simulink model "swim_12B_with_contracts_PP"  (R2019b)
settings: Solver=FixedStepDiscrete  StartTime=0.0  StopTime=10.0  FixedStep=0.200000  RelTol=1e-3  EnableMultiTasking=on
model workspace (MAT data in the model file):
  ContractValidatorBlocksMap = containers.Map
  ContractValidatorBlocksMap.serialization.keys = {'swim_12B_with_contracts/swim_12B_SWIMSpec/validator'}
  ContractValidatorBlocksMap.serialization.values{1}.block = 'swim_12B_with_contracts/swim_12B_SWIMSpec/validator'
  ContractValidatorBlocksMap.serialization.values{1}.assumePorts = 1
  ContractValidatorBlocksMap.serialization.values{1}.guaranteePorts = 3
  ContractValidatorBlocksMap.serialization.values{1}.modeBlocksPorts = 0
  ContractValidatorBlocksMap.serialization.values{1}.portHandles.Inport = [713.000976562 714.000976562 715.000976562 716.000976562]
  ContractValidatorBlocksMap.serialization.values{1}.portHandles.Outport = 717.000976562
  ContractValidatorBlocksMap.serialization.values{1}.portHandles.Enable = []
  ContractValidatorBlocksMap.serialization.values{1}.portHandles.Trigger = []
  ContractValidatorBlocksMap.serialization.values{1}.portHandles.State = []
  ContractValidatorBlocksMap.serialization.values{1}.portHandles.LConn = []
  ContractValidatorBlocksMap.serialization.values{1}.portHandles.RConn = []
  ContractValidatorBlocksMap.serialization.values{1}.portHandles.Ifaction = []
  ContractValidatorBlocksMap.serialization.values{1}.portHandles.Reset = []
  ContractValidatorBlocksMap.serialization.values{1}.portConnectivity(1).Type = '1'
  ContractValidatorBlocksMap.serialization.values{1}.portConnectivity(1).Position = [1210 730]
  ContractValidatorBlocksMap.serialization.values{1}.portConnectivity(1).SrcBlock = 336.034667969
  ContractValidatorBlocksMap.serialization.values{1}.portConnectivity(1).SrcPort = 0
  ContractValidatorBlocksMap.serialization.values{1}.portConnectivity(1).DstBlock = []
  ContractValidatorBlocksMap.serialization.values{1}.portConnectivity(1).DstPort = []
  ContractValidatorBlocksMap.serialization.values{1}.portConnectivity(2).Type = '2'
  ContractValidatorBlocksMap.serialization.values{1}.portConnectivity(2).Position = [1210 775]
  ContractValidatorBlocksMap.serialization.values{1}.portConnectivity(2).SrcBlock = 340.034667969
  ContractValidatorBlocksMap.serialization.values{1}.portConnectivity(2).SrcPort = 0
  ContractValidatorBlocksMap.serialization.values{1}.portConnectivity(2).DstBlock = []
  ContractValidatorBlocksMap.serialization.values{1}.portConnectivity(2).DstPort = []
  ContractValidatorBlocksMap.serialization.values{1}.portConnectivity(3).Type = '3'
  ContractValidatorBlocksMap.serialization.values{1}.portConnectivity(3).Position = [1210 820]
  ContractValidatorBlocksMap.serialization.values{1}.portConnectivity(3).SrcBlock = 344.034667969
  ContractValidatorBlocksMap.serialization.values{1}.portConnectivity(3).SrcPort = 0
  ContractValidatorBlocksMap.serialization.values{1}.portConnectivity(3).DstBlock = []
  ContractValidatorBlocksMap.serialization.values{1}.portConnectivity(3).DstPort = []
  ContractValidatorBlocksMap.serialization.values{1}.portConnectivity(4).Type = '4'
  ContractValidatorBlocksMap.serialization.values{1}.portConnectivity(4).Position = [1210 865]
  ContractValidatorBlocksMap.serialization.values{1}.portConnectivity(4).SrcBlock = 348.034667969
  ContractValidatorBlocksMap.serialization.values{1}.portConnectivity(4).SrcPort = 0
  ContractValidatorBlocksMap.serialization.values{1}.portConnectivity(4).DstBlock = []
  ContractValidatorBlocksMap.serialization.values{1}.portConnectivity(4).DstPort = []
  ContractValidatorBlocksMap.serialization.values{1}.portConnectivity(5).Type = '1'
  ContractValidatorBlocksMap.serialization.values{1}.portConnectivity(5).Position = [1250 800]
  ContractValidatorBlocksMap.serialization.values{1}.portConnectivity(5).SrcBlock = []
  ContractValidatorBlocksMap.serialization.values{1}.portConnectivity(5).SrcPort = []
  ContractValidatorBlocksMap.serialization.values{1}.portConnectivity(5).DstBlock = 379.034667969
  ContractValidatorBlocksMap.serialization.values{1}.portConnectivity(5).DstPort = 0
  ContractValidatorBlocksMap.serialization.uniformity = 0
  ContractValidatorBlocksMap.serialization.keyType = 'char'
  ContractValidatorBlocksMap.serialization.valueType = 'any'
  already_pp = 1
  compositionalMap.analysisNames = {'swim_12B_with_contracts_PP/swim_airspeed'}
  compositionalMap.compositionalOptions = {{''}}
  compositionalMap.selectedOptions = 1
  maskControlsMap = containers.Map
  maskControlsMap.serialization.keys = {'swim_12B_with_contracts_PP/swim_12B_SWIMSpec/SWIM_minus_002'}
  maskControlsMap.serialization.values = {{'Display_counter_example_as_signals', 'Display_counter_example_as_tables', 'Display_counter_example_as_HTML_tables', 'Generate_an_outer_model_for_the_counter_example', 'Generate_an_inner_model_for_the_counter_example'}}
  maskControlsMap.serialization.uniformity = 0
  maskControlsMap.serialization.keyType = 'char'
  maskControlsMap.serialization.valueType = 'any'
  nodeNameToBlockNameMap = containers.Map
  nodeNameToBlockNameMap.serialization.keys{1} = 'A_1'
  nodeNameToBlockNameMap.serialization.keys{2} = 'A_equal__equal__gt_B_1'
  nodeNameToBlockNameMap.serialization.keys{3} = 'AircraftWeight_lbs_1'
  nodeNameToBlockNameMap.serialization.keys{4} = 'AirspeedMonitoring_1'
  nodeNameToBlockNameMap.serialization.keys{5} = 'AirspeedMonitoring_435_035'
  nodeNameToBlockNameMap.serialization.keys{6} = 'B_1'
  nodeNameToBlockNameMap.serialization.keys{7} = 'CalculateminimumimpactpressureforAGCASoperationtobesuspendedandsenttostandby_1'
  nodeNameToBlockNameMap.serialization.keys{8} = 'CalculateminimumimpactpressureforAGCASoperationtobesuspendedandsenttostandby_495_035'
  nodeNameToBlockNameMap.serialization.keys{9} = 'CalculateminimumimpactpressureforwarningtopilotthatAGCASoperationisdegraded_1'
  nodeNameToBlockNameMap.serialization.keys{10} = 'CalculateminimumimpactpressureforwarningtopilotthatAGCASoperationisdegraded_503_035'
  nodeNameToBlockNameMap.serialization.keys{11} = 'CalculatetheminimumcalibratedairspeedbasedonCatSwitch_1'
  nodeNameToBlockNameMap.serialization.keys{12} = 'CalculatetheminimumcalibratedairspeedbasedonCatSwitch_519_002'
  nodeNameToBlockNameMap.serialization.keys{13} = 'Constant1_1'
  nodeNameToBlockNameMap.serialization.keys{14} = 'Constant2_1'
  nodeNameToBlockNameMap.serialization.keys{15} = 'Constant3_1'
  nodeNameToBlockNameMap.serialization.keys{16} = 'Constant4_1'
  nodeNameToBlockNameMap.serialization.keys{17} = 'Constant_1'
  nodeNameToBlockNameMap.serialization.keys{18} = 'E_AI_IMPACT_PRESSURE_1'
  nodeNameToBlockNameMap.serialization.keys{19} = 'Gain1_1'
  nodeNameToBlockNameMap.serialization.keys{20} = 'Gain_1'
  nodeNameToBlockNameMap.serialization.keys{21} = 'Gettheaircraftweight_1'
  nodeNameToBlockNameMap.serialization.keys{22} = 'Gettheaircraftweight_566_001'
  nodeNameToBlockNameMap.serialization.keys{23} = 'If1_1'
  nodeNameToBlockNameMap.serialization.keys{24} = 'If1_2'
  nodeNameToBlockNameMap.serialization.keys{25} = 'IfActionSubsystem1_1'
  nodeNameToBlockNameMap.serialization.keys{26} = 'IfActionSubsystem1_447_035'
  nodeNameToBlockNameMap.serialization.keys{27} = 'IfActionSubsystem1_537_018'
  nodeNameToBlockNameMap.serialization.keys{28} = 'IfActionSubsystem1_592_001'
  nodeNameToBlockNameMap.serialization.keys{29} = 'IfActionSubsystem1_608_001'
  nodeNameToBlockNameMap.serialization.keys{30} = 'IfActionSubsystem2_1'
  nodeNameToBlockNameMap.serialization.keys{31} = 'IfActionSubsystem2_452_035'
  nodeNameToBlockNameMap.serialization.keys{32} = 'IfActionSubsystem3_1'
  nodeNameToBlockNameMap.serialization.keys{33} = 'IfActionSubsystem3_457_035'
  nodeNameToBlockNameMap.serialization.keys{34} = 'IfActionSubsystem_1'
  nodeNameToBlockNameMap.serialization.keys{35} = 'IfActionSubsystem_442_035'
  nodeNameToBlockNameMap.serialization.keys{36} = 'IfActionSubsystem_524_002'
  nodeNameToBlockNameMap.serialization.keys{37} = 'IfActionSubsystem_582_001'
  nodeNameToBlockNameMap.serialization.keys{38} = 'IfActionSubsystem_587_001'
  nodeNameToBlockNameMap.serialization.keys{39} = 'If_1'
  nodeNameToBlockNameMap.serialization.keys{40} = 'If_2'
  nodeNameToBlockNameMap.serialization.keys{41} = 'In1_1'
  nodeNameToBlockNameMap.serialization.keys{42} = 'IssueWarning_1'
  nodeNameToBlockNameMap.serialization.keys{43} = 'IssueWarning_570_001'
  nodeNameToBlockNameMap.serialization.keys{44} = 'LogicalOperator1_1'
  nodeNameToBlockNameMap.serialization.keys{45} = 'LogicalOperator2_1'
  nodeNameToBlockNameMap.serialization.keys{46} = 'LogicalOperator_1'
  nodeNameToBlockNameMap.serialization.keys{47} = 'Logical_newline_Operator1_1'
  nodeNameToBlockNameMap.serialization.keys{48} = 'Logical_newline_Operator_1'
  nodeNameToBlockNameMap.serialization.keys{49} = 'Merge1_1'
  nodeNameToBlockNameMap.serialization.keys{50} = 'Merge_1'
  nodeNameToBlockNameMap.serialization.keys{51} = 'Out1_1'
  nodeNameToBlockNameMap.serialization.keys{52} = 'RelationalOperator1_1'
  nodeNameToBlockNameMap.serialization.keys{53} = 'RelationalOperator2_1'
  nodeNameToBlockNameMap.serialization.keys{54} = 'RelationalOperator3_1'
  nodeNameToBlockNameMap.serialization.keys{55} = 'RelationalOperator4_1'
  nodeNameToBlockNameMap.serialization.keys{56} = 'RelationalOperator_1'
  nodeNameToBlockNameMap.serialization.keys{57} = 'SWIMSpec_CalAirspeedMin_1'
  nodeNameToBlockNameMap.serialization.keys{58} = 'SWIMSpec_lowSpeedWarningAllowed_1'
  nodeNameToBlockNameMap.serialization.keys{59} = 'SWIMSpec_storeCat_1'
  nodeNameToBlockNameMap.serialization.keys{60} = 'SWIMSpec_swimGet_agcasLowSpeedWarn_1'
  nodeNameToBlockNameMap.serialization.keys{61} = 'SWIMSpec_vehAirPress_1'
  nodeNameToBlockNameMap.serialization.keys{62} = 'SWIMSpec_warningTrigForMinPress_1'
  nodeNameToBlockNameMap.serialization.keys{63} = 'SWIMSpec_weight_1'
  nodeNameToBlockNameMap.serialization.keys{64} = 'SWIM_ASWarningAllowed_1'
  nodeNameToBlockNameMap.serialization.keys{65} = 'SWIM_AirspeedWarningAllowed_1'
  nodeNameToBlockNameMap.serialization.keys{66} = 'SWIM_CalAirspeedmin_kts_1'
  nodeNameToBlockNameMap.serialization.keys{67} = 'SWIM_Qcmin_lbspft2_1'
  nodeNameToBlockNameMap.serialization.keys{68} = 'SWIM_SelfAgcasLowSpeedWarn_1'
  nodeNameToBlockNameMap.serialization.keys{69} = 'SWIM_minus_001A_1'
  nodeNameToBlockNameMap.serialization.keys{70} = 'SWIM_minus_001A_340_035'
  nodeNameToBlockNameMap.serialization.keys{71} = 'SWIM_minus_001B_1'
  nodeNameToBlockNameMap.serialization.keys{72} = 'SWIM_minus_001B_344_035'
  nodeNameToBlockNameMap.serialization.keys{73} = 'SWIM_minus_002_1'
  nodeNameToBlockNameMap.serialization.keys{74} = 'SWIM_minus_002_348_035'
  nodeNameToBlockNameMap.serialization.keys{75} = 'S_ImpactPressure_lbspft2_1'
  nodeNameToBlockNameMap.serialization.keys{76} = 'Sqrt_1'
  nodeNameToBlockNameMap.serialization.keys{77} = 'Sum1_1'
  nodeNameToBlockNameMap.serialization.keys{78} = 'Sum_1'
  nodeNameToBlockNameMap.serialization.keys{79} = 'UnitDelay_1'
  nodeNameToBlockNameMap.serialization.keys{80} = 'assume_1'
  nodeNameToBlockNameMap.serialization.keys{81} = 'assume_336_035'
  nodeNameToBlockNameMap.serialization.keys{82} = 'cvGet_V_AgcasLowSpeedWarn_1'
  nodeNameToBlockNameMap.serialization.keys{83} = 'diGet_S_CatSwitchPosition_1'
  nodeNameToBlockNameMap.serialization.keys{84} = 'diGet_S_LandingGearAltFlap_1'
  nodeNameToBlockNameMap.serialization.keys{85} = 'guarantee_1'
  nodeNameToBlockNameMap.serialization.keys{86} = 'lowSpeedWarningTrue_operator_1'
  nodeNameToBlockNameMap.serialization.keys{87} = 'muxGet_T_Mux_AircraftGrossWeight_lbs_1'
  nodeNameToBlockNameMap.serialization.keys{88} = 'muxGet_T_Mux_AirspeedMonitorEnable_1'
  nodeNameToBlockNameMap.serialization.keys{89} = 'o_SWIM_CalAirspeedmin_kts_1'
  nodeNameToBlockNameMap.serialization.keys{90} = 'o_SWIM_QcMinDisable_lbspft2_1'
  nodeNameToBlockNameMap.serialization.keys{91} = 'o_SWIM_Qcmin_lbspft2_1'
  nodeNameToBlockNameMap.serialization.keys{92} = 'olcGet_AgcasInterlocks_1'
  nodeNameToBlockNameMap.serialization.keys{93} = 'spec122_operator_1'
  nodeNameToBlockNameMap.serialization.keys{94} = 'spec122_rhs_2_1'
  nodeNameToBlockNameMap.serialization.keys{95} = 'spec139_operator_1'
  nodeNameToBlockNameMap.serialization.keys{96} = 'spec139_operator_355_035'
  nodeNameToBlockNameMap.serialization.keys{97} = 'spec156_operator_1'
  nodeNameToBlockNameMap.serialization.keys{98} = 'spec156_operator_356_035'
  nodeNameToBlockNameMap.serialization.keys{99} = 'spec170_operator_1'
  nodeNameToBlockNameMap.serialization.keys{100} = 'spec170_operator_357_035'
  nodeNameToBlockNameMap.serialization.keys{101} = 'sqrtOfWeight_sqrt_call_1'
  nodeNameToBlockNameMap.serialization.keys{102} = 'swimGet_AgcasLowSpeedWarn_1'
  nodeNameToBlockNameMap.serialization.keys{103} = 'swimGet_QcMinDisable_lbspft2_1'
  nodeNameToBlockNameMap.serialization.keys{104} = 'swim_12B_SWIMSpec_328_035'
  nodeNameToBlockNameMap.serialization.keys{105} = 'swim_12B_with_contracts_PP'
  nodeNameToBlockNameMap.serialization.keys{106} = 'swim_airspeed_1'
  nodeNameToBlockNameMap.serialization.keys{107} = 'swim_airspeed_2'
  nodeNameToBlockNameMap.serialization.keys{108} = 'swim_airspeed_3'
  nodeNameToBlockNameMap.serialization.keys{109} = 'swim_airspeed_4'
  nodeNameToBlockNameMap.serialization.keys{110} = 'swim_airspeed_427_035'
  nodeNameToBlockNameMap.serialization.keys{111} = 'swim_airspeed_5'
  nodeNameToBlockNameMap.serialization.keys{112} = 'valid_1'
  nodeNameToBlockNameMap.serialization.keys{113} = 'xxSWIMSpec_10_operator_1'
  nodeNameToBlockNameMap.serialization.keys{114} = 'xxSWIMSpec_11_operator_1'
  nodeNameToBlockNameMap.serialization.keys{115} = 'xxSWIMSpec_12_rhs_1'
  nodeNameToBlockNameMap.serialization.keys{116} = 'xxSWIMSpec_13_rhs_1'
  nodeNameToBlockNameMap.serialization.keys{117} = 'xxSWIMSpec_14_rhs_1'
  nodeNameToBlockNameMap.serialization.keys{118} = 'xxSWIMSpec_1_operator_1'
  nodeNameToBlockNameMap.serialization.keys{119} = 'xxSWIMSpec_2_operator_1'
  nodeNameToBlockNameMap.serialization.keys{120} = 'xxSWIMSpec_2_rhs_2_1'
  nodeNameToBlockNameMap.serialization.keys{121} = 'xxSWIMSpec_3_operator_1'
  nodeNameToBlockNameMap.serialization.keys{122} = 'xxSWIMSpec_4_operator_1'
  nodeNameToBlockNameMap.serialization.keys{123} = 'xxSWIMSpec_4_rhs_1_1'
  nodeNameToBlockNameMap.serialization.keys{124} = 'xxSWIMSpec_5_operator_1'
  nodeNameToBlockNameMap.serialization.keys{125} = 'xxSWIMSpec_5_rhs_2_1'
  nodeNameToBlockNameMap.serialization.keys{126} = 'xxSWIMSpec_6_operator_1'
  nodeNameToBlockNameMap.serialization.keys{127} = 'xxSWIMSpec_7_operator_1'
  nodeNameToBlockNameMap.serialization.keys{128} = 'xxSWIMSpec_8_operator_1'
  nodeNameToBlockNameMap.serialization.keys{129} = 'xxSWIMSpec_8_rhs_1_1'
  nodeNameToBlockNameMap.serialization.keys{130} = 'xxSWIMSpec_9_operator_1'
  nodeNameToBlockNameMap.serialization.keys{131} = 'xxSWIMSpec_9_rhs_2_1'
  nodeNameToBlockNameMap.serialization.values{1} = 'swim_12B_with_contracts_PP/swim_12B_SWIMSpec/spec170_operator/A'
  nodeNameToBlockNameMap.serialization.values{2} = 'swim_12B_with_contracts_PP/swim_12B_SWIMSpec/spec170_operator/A_equal__equal__gt_B'
  nodeNameToBlockNameMap.serialization.values{3} = 'swim_12B_with_contracts_PP/swim_airspeed/Gettheaircraftweight/AircraftWeight_lbs'
  nodeNameToBlockNameMap.serialization.values{4} = 'swim_12B_with_contracts_PP/swim_airspeed/AirspeedMonitoring'
  nodeNameToBlockNameMap.serialization.values{5} = 'swim_12B_with_contracts_PP/swim_airspeed/AirspeedMonitoring'
  nodeNameToBlockNameMap.serialization.values{6} = 'swim_12B_with_contracts_PP/swim_12B_SWIMSpec/spec170_operator/B'
  nodeNameToBlockNameMap.serialization.values{7} = 'swim_12B_with_contracts_PP/swim_airspeed/CalculateminimumimpactpressureforAGCASoperationtobesuspendedandsenttostandby'
  nodeNameToBlockNameMap.serialization.values{8} = 'swim_12B_with_contracts_PP/swim_airspeed/CalculateminimumimpactpressureforAGCASoperationtobesuspendedandsenttostandby'
  nodeNameToBlockNameMap.serialization.values{9} = 'swim_12B_with_contracts_PP/swim_airspeed/CalculateminimumimpactpressureforwarningtopilotthatAGCASoperationisdegraded'
  nodeNameToBlockNameMap.serialization.values{10} = 'swim_12B_with_contracts_PP/swim_airspeed/CalculateminimumimpactpressureforwarningtopilotthatAGCASoperationisdegraded'
  nodeNameToBlockNameMap.serialization.values{11} = 'swim_12B_with_contracts_PP/swim_airspeed/CalculatetheminimumcalibratedairspeedbasedonCatSwitch'
  nodeNameToBlockNameMap.serialization.values{12} = 'swim_12B_with_contracts_PP/swim_airspeed/CalculatetheminimumcalibratedairspeedbasedonCatSwitch'
  nodeNameToBlockNameMap.serialization.values{13} = 'swim_12B_with_contracts_PP/swim_airspeed/IssueWarning/Constant1'
  nodeNameToBlockNameMap.serialization.values{14} = 'swim_12B_with_contracts_PP/swim_airspeed/IssueWarning/Constant2'
  nodeNameToBlockNameMap.serialization.values{15} = 'swim_12B_with_contracts_PP/swim_airspeed/IssueWarning/Constant3'
  nodeNameToBlockNameMap.serialization.values{16} = 'swim_12B_with_contracts_PP/swim_airspeed/IssueWarning/Constant4'
  nodeNameToBlockNameMap.serialization.values{17} = 'swim_12B_with_contracts_PP/swim_airspeed/IssueWarning/IfActionSubsystem/IfActionSubsystem1/Constant'
  nodeNameToBlockNameMap.serialization.values{18} = 'swim_12B_with_contracts_PP/E_AI_IMPACT_PRESSURE'
  nodeNameToBlockNameMap.serialization.values{19} = 'swim_12B_with_contracts_PP/swim_airspeed/CalculateminimumimpactpressureforwarningtopilotthatAGCASoperationisdegraded/Gain1'
  nodeNameToBlockNameMap.serialization.values{20} = 'swim_12B_with_contracts_PP/swim_airspeed/CalculatetheminimumcalibratedairspeedbasedonCatSwitch/IfActionSubsystem1/Gain'
  nodeNameToBlockNameMap.serialization.values{21} = 'swim_12B_with_contracts_PP/swim_airspeed/Gettheaircraftweight'
  nodeNameToBlockNameMap.serialization.values{22} = 'swim_12B_with_contracts_PP/swim_airspeed/Gettheaircraftweight'
  nodeNameToBlockNameMap.serialization.values{23} = 'swim_12B_with_contracts_PP/swim_airspeed/AirspeedMonitoring/If1'
  nodeNameToBlockNameMap.serialization.values{24} = 'swim_12B_with_contracts_PP/swim_airspeed/AirspeedMonitoring/If1'
  nodeNameToBlockNameMap.serialization.values{25} = 'swim_12B_with_contracts_PP/swim_airspeed/IssueWarning/IfActionSubsystem1'
  nodeNameToBlockNameMap.serialization.values{26} = 'swim_12B_with_contracts_PP/swim_airspeed/AirspeedMonitoring/IfActionSubsystem1'
  nodeNameToBlockNameMap.serialization.values{27} = 'swim_12B_with_contracts_PP/swim_airspeed/CalculatetheminimumcalibratedairspeedbasedonCatSwitch/IfActionSubsystem1'
  nodeNameToBlockNameMap.serialization.values{28} = 'swim_12B_with_contracts_PP/swim_airspeed/IssueWarning/IfActionSubsystem/IfActionSubsystem1'
  nodeNameToBlockNameMap.serialization.values{29} = 'swim_12B_with_contracts_PP/swim_airspeed/IssueWarning/IfActionSubsystem1'
  nodeNameToBlockNameMap.serialization.values{30} = 'swim_12B_with_contracts_PP/swim_airspeed/AirspeedMonitoring/IfActionSubsystem2'
  nodeNameToBlockNameMap.serialization.values{31} = 'swim_12B_with_contracts_PP/swim_airspeed/AirspeedMonitoring/IfActionSubsystem2'
  nodeNameToBlockNameMap.serialization.values{32} = 'swim_12B_with_contracts_PP/swim_airspeed/AirspeedMonitoring/IfActionSubsystem3'
  nodeNameToBlockNameMap.serialization.values{33} = 'swim_12B_with_contracts_PP/swim_airspeed/AirspeedMonitoring/IfActionSubsystem3'
  nodeNameToBlockNameMap.serialization.values{34} = 'swim_12B_with_contracts_PP/swim_airspeed/IssueWarning/IfActionSubsystem'
  nodeNameToBlockNameMap.serialization.values{35} = 'swim_12B_with_contracts_PP/swim_airspeed/AirspeedMonitoring/IfActionSubsystem'
  nodeNameToBlockNameMap.serialization.values{36} = 'swim_12B_with_contracts_PP/swim_airspeed/CalculatetheminimumcalibratedairspeedbasedonCatSwitch/IfActionSubsystem'
  nodeNameToBlockNameMap.serialization.values{37} = 'swim_12B_with_contracts_PP/swim_airspeed/IssueWarning/IfActionSubsystem'
  nodeNameToBlockNameMap.serialization.values{38} = 'swim_12B_with_contracts_PP/swim_airspeed/IssueWarning/IfActionSubsystem/IfActionSubsystem'
  nodeNameToBlockNameMap.serialization.values{39} = 'swim_12B_with_contracts_PP/swim_airspeed/IssueWarning/If'
  nodeNameToBlockNameMap.serialization.values{40} = 'swim_12B_with_contracts_PP/swim_airspeed/IssueWarning/If'
  nodeNameToBlockNameMap.serialization.values{41} = 'swim_12B_with_contracts_PP/swim_airspeed/IssueWarning/IfActionSubsystem1/In1'
  nodeNameToBlockNameMap.serialization.values{42} = 'swim_12B_with_contracts_PP/swim_airspeed/IssueWarning'
  nodeNameToBlockNameMap.serialization.values{43} = 'swim_12B_with_contracts_PP/swim_airspeed/IssueWarning'
  nodeNameToBlockNameMap.serialization.values{44} = 'swim_12B_with_contracts_PP/swim_airspeed/IssueWarning/LogicalOperator1'
  nodeNameToBlockNameMap.serialization.values{45} = 'swim_12B_with_contracts_PP/swim_airspeed/IssueWarning/LogicalOperator2'
  nodeNameToBlockNameMap.serialization.values{46} = 'swim_12B_with_contracts_PP/swim_airspeed/AirspeedMonitoring/LogicalOperator'
  nodeNameToBlockNameMap.serialization.values{47} = 'swim_12B_with_contracts_PP/swim_12B_SWIMSpec/spec170_operator/Logical_newline_Operator1'
  nodeNameToBlockNameMap.serialization.values{48} = 'swim_12B_with_contracts_PP/swim_12B_SWIMSpec/spec170_operator/Logical_newline_Operator'
  nodeNameToBlockNameMap.serialization.values{49} = 'swim_12B_with_contracts_PP/swim_airspeed/AirspeedMonitoring/Merge1'
  nodeNameToBlockNameMap.serialization.values{50} = 'swim_12B_with_contracts_PP/swim_airspeed/IssueWarning/Merge'
  nodeNameToBlockNameMap.serialization.values{51} = 'swim_12B_with_contracts_PP/swim_airspeed/IssueWarning/IfActionSubsystem1/Out1'
  nodeNameToBlockNameMap.serialization.values{52} = 'swim_12B_with_contracts_PP/swim_airspeed/IssueWarning/RelationalOperator1'
  nodeNameToBlockNameMap.serialization.values{53} = 'swim_12B_with_contracts_PP/swim_airspeed/IssueWarning/RelationalOperator2'
  nodeNameToBlockNameMap.serialization.values{54} = 'swim_12B_with_contracts_PP/swim_airspeed/IssueWarning/RelationalOperator3'
  nodeNameToBlockNameMap.serialization.values{55} = 'swim_12B_with_contracts_PP/swim_airspeed/IssueWarning/RelationalOperator4'
  nodeNameToBlockNameMap.serialization.values{56} = 'swim_12B_with_contracts_PP/swim_airspeed/IssueWarning/IfActionSubsystem/RelationalOperator'
  nodeNameToBlockNameMap.serialization.values{57} = 'swim_12B_with_contracts_PP/swim_12B_SWIMSpec/SWIMSpec_CalAirspeedMin'
  nodeNameToBlockNameMap.serialization.values{58} = 'swim_12B_with_contracts_PP/swim_12B_SWIMSpec/SWIMSpec_lowSpeedWarningAllowed'
  nodeNameToBlockNameMap.serialization.values{59} = 'swim_12B_with_contracts_PP/swim_12B_SWIMSpec/SWIMSpec_storeCat'
  nodeNameToBlockNameMap.serialization.values{60} = 'swim_12B_with_contracts_PP/swim_12B_SWIMSpec/SWIMSpec_swimGet_agcasLowSpeedWarn'
  nodeNameToBlockNameMap.serialization.values{61} = 'swim_12B_with_contracts_PP/swim_12B_SWIMSpec/SWIMSpec_vehAirPress'
  nodeNameToBlockNameMap.serialization.values{62} = 'swim_12B_with_contracts_PP/swim_12B_SWIMSpec/SWIMSpec_warningTrigForMinPress'
  nodeNameToBlockNameMap.serialization.values{63} = 'swim_12B_with_contracts_PP/swim_12B_SWIMSpec/SWIMSpec_weight'
  nodeNameToBlockNameMap.serialization.values{64} = 'swim_12B_with_contracts_PP/SWIM_ASWarningAllowed'
  nodeNameToBlockNameMap.serialization.values{65} = 'swim_12B_with_contracts_PP/swim_airspeed/IssueWarning/SWIM_AirspeedWarningAllowed'
  nodeNameToBlockNameMap.serialization.values{66} = 'swim_12B_with_contracts_PP/SWIM_CalAirspeedmin_kts'
  nodeNameToBlockNameMap.serialization.values{67} = 'swim_12B_with_contracts_PP/SWIM_Qcmin_lbspft2'
  nodeNameToBlockNameMap.serialization.values{68} = 'swim_12B_with_contracts_PP/swim_airspeed/IssueWarning/SWIM_SelfAgcasLowSpeedWarn'
  nodeNameToBlockNameMap.serialization.values{69} = 'swim_12B_with_contracts_PP/swim_12B_SWIMSpec/SWIM_minus_001A'
  nodeNameToBlockNameMap.serialization.values{70} = 'swim_12B_with_contracts_PP/swim_12B_SWIMSpec/SWIM_minus_001A'
  nodeNameToBlockNameMap.serialization.values{71} = 'swim_12B_with_contracts_PP/swim_12B_SWIMSpec/SWIM_minus_001B'
  nodeNameToBlockNameMap.serialization.values{72} = 'swim_12B_with_contracts_PP/swim_12B_SWIMSpec/SWIM_minus_001B'
  nodeNameToBlockNameMap.serialization.values{73} = 'swim_12B_with_contracts_PP/swim_12B_SWIMSpec/SWIM_minus_002'
  nodeNameToBlockNameMap.serialization.values{74} = 'swim_12B_with_contracts_PP/swim_12B_SWIMSpec/SWIM_minus_002'
  nodeNameToBlockNameMap.serialization.values{75} = 'swim_12B_with_contracts_PP/swim_airspeed/IssueWarning/S_ImpactPressure_lbspft2'
  nodeNameToBlockNameMap.serialization.values{76} = 'swim_12B_with_contracts_PP/swim_airspeed/CalculatetheminimumcalibratedairspeedbasedonCatSwitch/IfActionSubsystem1/Sqrt'
  nodeNameToBlockNameMap.serialization.values{77} = 'swim_12B_with_contracts_PP/swim_airspeed/CalculateminimumimpactpressureforwarningtopilotthatAGCASoperationisdegraded/Sum1'
  nodeNameToBlockNameMap.serialization.values{78} = 'swim_12B_with_contracts_PP/swim_airspeed/CalculatetheminimumcalibratedairspeedbasedonCatSwitch/IfActionSubsystem1/Sum'
  nodeNameToBlockNameMap.serialization.values{79} = 'swim_12B_with_contracts_PP/swim_airspeed/IssueWarning/UnitDelay'
  nodeNameToBlockNameMap.serialization.values{80} = 'swim_12B_with_contracts_PP/swim_12B_SWIMSpec/assume'
  nodeNameToBlockNameMap.serialization.values{81} = 'swim_12B_with_contracts_PP/swim_12B_SWIMSpec/assume'
  nodeNameToBlockNameMap.serialization.values{82} = 'swim_12B_with_contracts_PP/cvGet_V_AgcasLowSpeedWarn'
  nodeNameToBlockNameMap.serialization.values{83} = 'swim_12B_with_contracts_PP/diGet_S_CatSwitchPosition'
  nodeNameToBlockNameMap.serialization.values{84} = 'swim_12B_with_contracts_PP/diGet_S_LandingGearAltFlap'
  nodeNameToBlockNameMap.serialization.values{85} = 'swim_12B_with_contracts_PP/swim_12B_SWIMSpec/SWIM_minus_002/guarantee'
  nodeNameToBlockNameMap.serialization.values{86} = 'swim_12B_with_contracts_PP/swim_12B_SWIMSpec/lowSpeedWarningTrue_operator'
  nodeNameToBlockNameMap.serialization.values{87} = 'swim_12B_with_contracts_PP/muxGet_T_Mux_AircraftGrossWeight_lbs'
  nodeNameToBlockNameMap.serialization.values{88} = 'swim_12B_with_contracts_PP/muxGet_T_Mux_AirspeedMonitorEnable'
  nodeNameToBlockNameMap.serialization.values{89} = 'swim_12B_with_contracts_PP/swim_airspeed/CalculatetheminimumcalibratedairspeedbasedonCatSwitch/IfActionSubsystem1/o_SWIM_CalAirspeedmin_kts'
  nodeNameToBlockNameMap.serialization.values{90} = 'swim_12B_with_contracts_PP/swim_airspeed/CalculateminimumimpactpressureforAGCASoperationtobesuspendedandsenttostandby/o_SWIM_QcMinDisable_lbspft2'
  nodeNameToBlockNameMap.serialization.values{91} = 'swim_12B_with_contracts_PP/swim_airspeed/CalculateminimumimpactpressureforwarningtopilotthatAGCASoperationisdegraded/o_SWIM_Qcmin_lbspft2'
  nodeNameToBlockNameMap.serialization.values{92} = 'swim_12B_with_contracts_PP/olcGet_AgcasInterlocks'
  nodeNameToBlockNameMap.serialization.values{93} = 'swim_12B_with_contracts_PP/swim_12B_SWIMSpec/spec122_operator'
  nodeNameToBlockNameMap.serialization.values{94} = 'swim_12B_with_contracts_PP/swim_12B_SWIMSpec/spec122_rhs_2'
  nodeNameToBlockNameMap.serialization.values{95} = 'swim_12B_with_contracts_PP/swim_12B_SWIMSpec/spec139_operator'
  nodeNameToBlockNameMap.serialization.values{96} = 'swim_12B_with_contracts_PP/swim_12B_SWIMSpec/spec139_operator'
  nodeNameToBlockNameMap.serialization.values{97} = 'swim_12B_with_contracts_PP/swim_12B_SWIMSpec/spec156_operator'
  nodeNameToBlockNameMap.serialization.values{98} = 'swim_12B_with_contracts_PP/swim_12B_SWIMSpec/spec156_operator'
  nodeNameToBlockNameMap.serialization.values{99} = 'swim_12B_with_contracts_PP/swim_12B_SWIMSpec/spec170_operator'
  nodeNameToBlockNameMap.serialization.values{100} = 'swim_12B_with_contracts_PP/swim_12B_SWIMSpec/spec170_operator'
  nodeNameToBlockNameMap.serialization.values{101} = 'swim_12B_with_contracts_PP/swim_12B_SWIMSpec/sqrtOfWeight_sqrt_call'
  nodeNameToBlockNameMap.serialization.values{102} = 'swim_12B_with_contracts_PP/swimGet_AgcasLowSpeedWarn'
  nodeNameToBlockNameMap.serialization.values{103} = 'swim_12B_with_contracts_PP/swimGet_QcMinDisable_lbspft2'
  nodeNameToBlockNameMap.serialization.values{104} = 'swim_12B_with_contracts_PP/swim_12B_SWIMSpec/assume'
  nodeNameToBlockNameMap.serialization.values{105} = 'swim_12B_with_contracts_PP'
  nodeNameToBlockNameMap.serialization.values{106} = 'swim_12B_with_contracts_PP/swim_airspeed'
  nodeNameToBlockNameMap.serialization.values{107} = 'swim_12B_with_contracts_PP/swim_airspeed'
  nodeNameToBlockNameMap.serialization.values{108} = 'swim_12B_with_contracts_PP/swim_airspeed'
  nodeNameToBlockNameMap.serialization.values{109} = 'swim_12B_with_contracts_PP/swim_airspeed'
  nodeNameToBlockNameMap.serialization.values{110} = 'swim_12B_with_contracts_PP/swim_airspeed'
  nodeNameToBlockNameMap.serialization.values{111} = 'swim_12B_with_contracts_PP/swim_airspeed'
  nodeNameToBlockNameMap.serialization.values{112} = 'swim_12B_with_contracts_PP/swim_12B_SWIMSpec/valid'
  nodeNameToBlockNameMap.serialization.values{113} = 'swim_12B_with_contracts_PP/swim_12B_SWIMSpec/xxSWIMSpec_10_operator'
  nodeNameToBlockNameMap.serialization.values{114} = 'swim_12B_with_contracts_PP/swim_12B_SWIMSpec/xxSWIMSpec_11_operator'
  nodeNameToBlockNameMap.serialization.values{115} = 'swim_12B_with_contracts_PP/swim_12B_SWIMSpec/xxSWIMSpec_12_rhs'
  nodeNameToBlockNameMap.serialization.values{116} = 'swim_12B_with_contracts_PP/swim_12B_SWIMSpec/xxSWIMSpec_13_rhs'
  nodeNameToBlockNameMap.serialization.values{117} = 'swim_12B_with_contracts_PP/swim_12B_SWIMSpec/xxSWIMSpec_14_rhs'
  nodeNameToBlockNameMap.serialization.values{118} = 'swim_12B_with_contracts_PP/swim_12B_SWIMSpec/xxSWIMSpec_1_operator'
  nodeNameToBlockNameMap.serialization.values{119} = 'swim_12B_with_contracts_PP/swim_12B_SWIMSpec/xxSWIMSpec_2_operator'
  nodeNameToBlockNameMap.serialization.values{120} = 'swim_12B_with_contracts_PP/swim_12B_SWIMSpec/xxSWIMSpec_2_rhs_2'
  nodeNameToBlockNameMap.serialization.values{121} = 'swim_12B_with_contracts_PP/swim_12B_SWIMSpec/xxSWIMSpec_3_operator'
  nodeNameToBlockNameMap.serialization.values{122} = 'swim_12B_with_contracts_PP/swim_12B_SWIMSpec/xxSWIMSpec_4_operator'
  nodeNameToBlockNameMap.serialization.values{123} = 'swim_12B_with_contracts_PP/swim_12B_SWIMSpec/xxSWIMSpec_4_rhs_1'
  nodeNameToBlockNameMap.serialization.values{124} = 'swim_12B_with_contracts_PP/swim_12B_SWIMSpec/xxSWIMSpec_5_operator'
  nodeNameToBlockNameMap.serialization.values{125} = 'swim_12B_with_contracts_PP/swim_12B_SWIMSpec/xxSWIMSpec_5_rhs_2'
  nodeNameToBlockNameMap.serialization.values{126} = 'swim_12B_with_contracts_PP/swim_12B_SWIMSpec/xxSWIMSpec_6_operator'
  nodeNameToBlockNameMap.serialization.values{127} = 'swim_12B_with_contracts_PP/swim_12B_SWIMSpec/xxSWIMSpec_7_operator'
  nodeNameToBlockNameMap.serialization.values{128} = 'swim_12B_with_contracts_PP/swim_12B_SWIMSpec/xxSWIMSpec_8_operator'
  nodeNameToBlockNameMap.serialization.values{129} = 'swim_12B_with_contracts_PP/swim_12B_SWIMSpec/xxSWIMSpec_8_rhs_1'
  nodeNameToBlockNameMap.serialization.values{130} = 'swim_12B_with_contracts_PP/swim_12B_SWIMSpec/xxSWIMSpec_9_operator'
  nodeNameToBlockNameMap.serialization.values{131} = 'swim_12B_with_contracts_PP/swim_12B_SWIMSpec/xxSWIMSpec_9_rhs_2'
  nodeNameToBlockNameMap.serialization.uniformity = 1
  nodeNameToBlockNameMap.serialization.keyType = 'char'
  nodeNameToBlockNameMap.serialization.valueType = 'char'
  verificationResults : object (value not decoded)
undefined symbols (not defined in the file): contractAfterSimulation, ContractAssumeBlock, contractBeforeSimulation, ContractBlock, ContractGuaranteeBlock, ContractValidatorBlock, E_DI_CATI, E_DI_DOWN_OR_LOCKED, E_DI_UP_AND_NORMAL, E_MUX_ENABLED, E_OLC_INTERLOCK_NOT_FAILED, E_SWIM_ALLOWED, E_SWIM_NOT_ALLOWED, E_SWIM_WARNING_OFF, E_SWIM_WARNING_ON, saveValidatorParameters
settings Model: Creator=belottr  LastModifiedBy=hbourbou
settings DataIOCC: LimitDataPoints=on  SaveFormat=Array  ReturnWorkspaceOutputs=off
settings OptimizationCC: DefaultParameterBehavior=Inlined  ExpressionDepthLimit=2147483647  LifeSpan=inf
settings DebuggingCC: AlgebraicLoopMsg=error  ArtificialAlgebraicLoopMsg=error  UnderspecifiedInitializationDetection=Classic  MergeDetectMultiDrivingBlocksExec=none  SolverPrmCheckMsg=warning  SingleTaskRateTransMsg=error  StateNameClashWarn=warning  SFUnexpectedBacktrackingDiag=warning  SFNoUnconditionalDefaultTransitionDiag=warning  SFExecutionAtInitializationDiag=none  ArithmeticOperatorsInVariantConditions=warning
settings HardwareCC: ProdBitPerPointer=32  ProdBitPerSizeT=32  ProdBitPerPtrDiffT=32  ProdLargestAtomicFloat=None  ProdIntDivRoundTo=Undefined  ProdEndianess=Unspecified  ProdWordSize=32  ProdHWDeviceType=32-bit Generic
settings ModelReferenceCC: UpdateModelReferenceTargets=IfOutOfDate  PropagateSignalLabelsOutOfModel=off
settings SFSimCC: SimUseLocalCustomCode=off  CustomCodeUndefinedFunction=UseInterfaceOnly
settings RTWCC: RTWUseLocalCustomCode=off
settings CodeAppCC: StateflowObjectComments=on
settings GRTTargetCC: TargetLangStandard=C89/C90 (ANSI)  GeneratePreprocessorConditionals=Disable all
settings ConfigComp: CovMetricSettings=dw  CovHtmlReporting=on  CovSaveCumulativeToWorkspaceVar=on  CovSaveSingleToWorkspaceVar=on  CovExternalEMLEnable=off

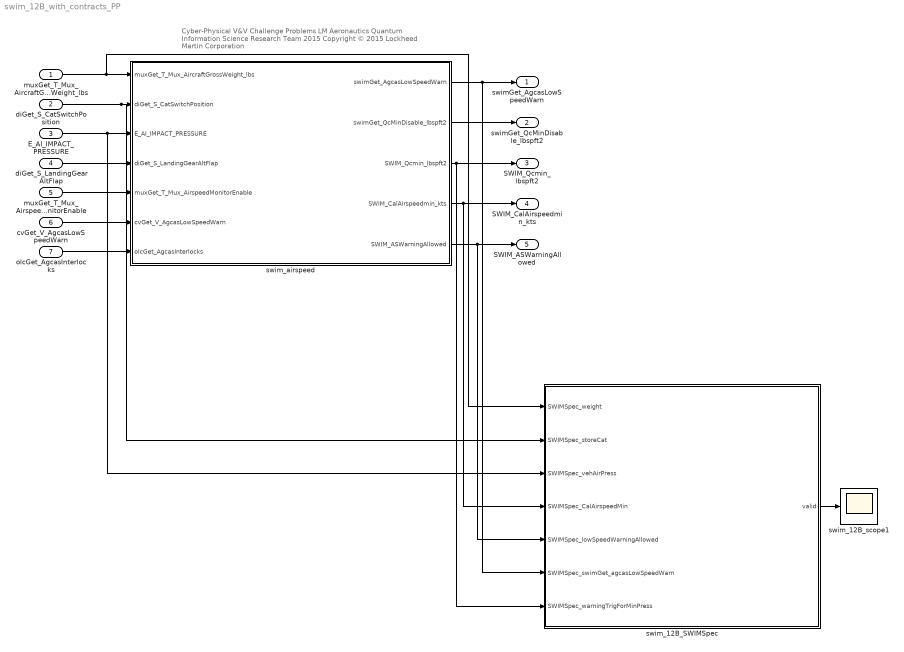
== system swim_12B_with_contracts_PP ==
  note: Cyber-Physical V&V Challenge Problems
      | LM Aeronautics Quantum Information Science Research Team 2015
      | Copyright © 2015 Lockheed Martin Corporation
  muxGet_T_Mux_AircraftGrossWeight_lbs : Inport  OutDataTypeStr=double
  diGet_S_CatSwitchPosition : Inport  Port=2  OutDataTypeStr=int32
  E_AI_IMPACT_PRESSURE : Inport  Port=3  OutDataTypeStr=double
  diGet_S_LandingGearAltFlap : Inport  Port=4  OutDataTypeStr=boolean
  muxGet_T_Mux_AirspeedMonitorEnable : Inport  Port=5  OutDataTypeStr=boolean
  cvGet_V_AgcasLowSpeedWarn : Inport  Port=6  OutDataTypeStr=boolean
  olcGet_AgcasInterlocks : Inport  Port=7  OutDataTypeStr=boolean
  swim_12B_SWIMSpec : Subsystem  TreatAsAtomicUnit=on  mask(ContractBlock){ContractBlockType=ContractBlock}
      mask init:
      | set_param(gcb, 'LinkStatus', 'none');
      mask DialogControl DescTextVar Prompt: Contract block
      mask Display:
      | text(0.5, 0.5, '{\bf\fontsize{20}Contract}', 'hor', 'center', 'texmode','on');
      | blocks = find_system(gcb, 'LookUnderMasks','all', 'SearchDepth',1,'BlockType','Inport');
      | for i = 1 : length(blocks)
      |     blockName = get_param(blocks(i), 'Name');
      |     [path, blockName] = fileparts(char(blockName));
      |     port_label('input', i, blockName);
      | end
      | 
      | blocks = find_system(gcb, 'LookUnderMasks','all', 'SearchDepth',1,'BlockType','Outport');
      | for i = 1 : length(blocks)
      |     blockName = get_param(blocks(i), 'Name');
      |     [path, blockName] = fileparts(char(blockName));
      |     port_label('output', i, blockName);
      | end
  swim_12B_scope1 : Scope
  swim_airspeed : Subsystem  TreatAsAtomicUnit=on
  swimGet_AgcasLowSpeedWarn : Outport  VectorParamsAs1DForOutWhenUnconnected=off
  swimGet_QcMinDisable_lbspft2 : Outport  Port=2  VectorParamsAs1DForOutWhenUnconnected=off
  SWIM_Qcmin_lbspft2 : Outport  Port=3  VectorParamsAs1DForOutWhenUnconnected=off
  SWIM_CalAirspeedmin_kts : Outport  Port=4  VectorParamsAs1DForOutWhenUnconnected=off
  SWIM_ASWarningAllowed : Outport  Port=5  VectorParamsAs1DForOutWhenUnconnected=off
  wires:
  muxGet_T_Mux_AircraftGrossWeight_lbs/1 -> swim_airspeed/1(muxGet_T_Mux_AircraftGrossWeight_lbs), swim_12B_SWIMSpec/1(SWIMSpec_weight)
  diGet_S_CatSwitchPosition/1 -> swim_airspeed/2(diGet_S_CatSwitchPosition), swim_12B_SWIMSpec/2(SWIMSpec_storeCat)
  E_AI_IMPACT_PRESSURE/1 -> swim_airspeed/3(E_AI_IMPACT_PRESSURE), swim_12B_SWIMSpec/3(SWIMSpec_vehAirPress)
  diGet_S_LandingGearAltFlap/1 -> swim_airspeed/4(diGet_S_LandingGearAltFlap)
  muxGet_T_Mux_AirspeedMonitorEnable/1 -> swim_airspeed/5(muxGet_T_Mux_AirspeedMonitorEnable)
  cvGet_V_AgcasLowSpeedWarn/1 -> swim_airspeed/6(cvGet_V_AgcasLowSpeedWarn)
  olcGet_AgcasInterlocks/1 -> swim_airspeed/7(olcGet_AgcasInterlocks)
  swim_airspeed/3(SWIM_Qcmin_lbspft2) -> SWIM_Qcmin_lbspft2/1, swim_12B_SWIMSpec/7(SWIMSpec_warningTrigForMinPress)
  swim_airspeed/2(swimGet_QcMinDisable_lbspft2) -> swimGet_QcMinDisable_lbspft2/1
  swim_airspeed/1(swimGet_AgcasLowSpeedWarn) -> swim_12B_SWIMSpec/6(SWIMSpec_swimGet_agcasLowSpeedWarn), swimGet_AgcasLowSpeedWarn/1
  swim_airspeed/4(SWIM_CalAirspeedmin_kts) -> SWIM_CalAirspeedmin_kts/1, swim_12B_SWIMSpec/4(SWIMSpec_CalAirspeedMin)
  swim_airspeed/5(SWIM_ASWarningAllowed) -> SWIM_ASWarningAllowed/1, swim_12B_SWIMSpec/5(SWIMSpec_lowSpeedWarningAllowed)
  swim_12B_SWIMSpec/1(valid) -> swim_12B_scope1/1

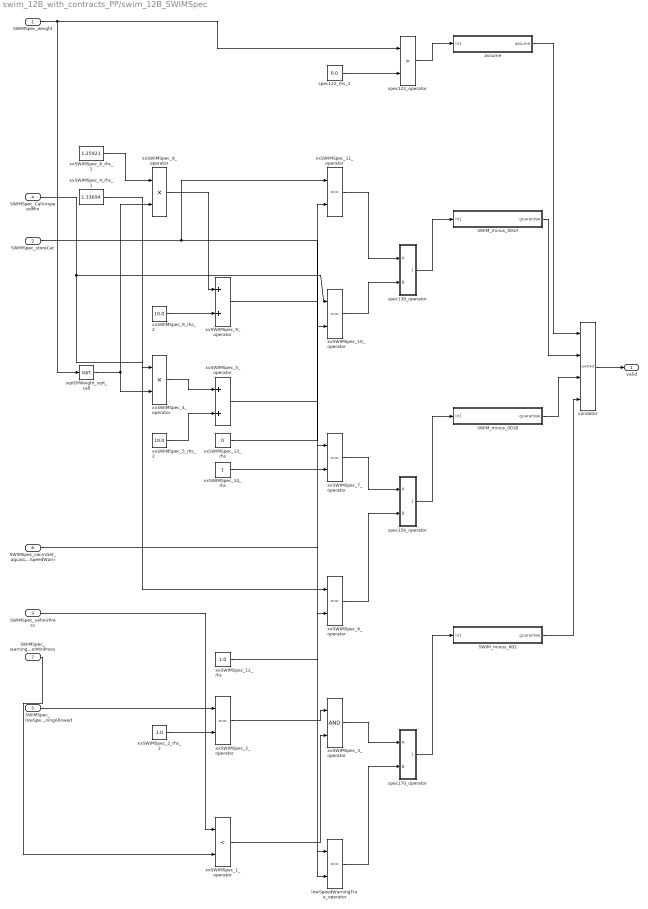
== system swim_12B_with_contracts_PP/swim_12B_SWIMSpec ==
  SWIMSpec_weight : Inport  OutDataTypeStr=double
  SWIMSpec_storeCat : Inport  Port=2
  SWIMSpec_vehAirPress : Inport  Port=3  OutDataTypeStr=double
  SWIMSpec_CalAirspeedMin : Inport  Port=4  OutDataTypeStr=double
  SWIMSpec_lowSpeedWarningAllowed : Inport  Port=5  OutDataTypeStr=double
  SWIMSpec_swimGet_agcasLowSpeedWarn : Inport  Port=6  OutDataTypeStr=double
  SWIMSpec_warningTrigForMinPress : Inport  Port=7  OutDataTypeStr=double
  SWIM_minus_001A : Subsystem  TreatAsAtomicUnit=on  mask(ContractGuaranteeBlock){ContractBlockType=ContractGuaranteeBlock}
      mask init:
      | set_param(gcb, 'LinkStatus', 'none');
      mask DialogControl DescTextVar Prompt: Guarantee block
  SWIM_minus_001B : Subsystem  TreatAsAtomicUnit=on  mask(ContractGuaranteeBlock){ContractBlockType=ContractGuaranteeBlock}
      mask init:
      | set_param(gcb, 'LinkStatus', 'none');
      mask DialogControl DescTextVar Prompt: Guarantee block
  SWIM_minus_002 : Subsystem  TreatAsAtomicUnit=on  mask(ContractGuaranteeBlock){ContractBlockType=ContractGuaranteeBlock}
      mask init:
      | set_param(gcb, 'LinkStatus', 'none');
      mask DialogControl DescTextVar Prompt: Guarantee block
      mask DialogControl Display_counter_example_as_signals Prompt: Display counter example as signals
      mask DialogControl Display_counter_example_as_signals Callback: displayCexSignals(1, 1);
      mask DialogControl Display_counter_example_as_tables Prompt: Display counter example as tables
      mask DialogControl Display_counter_example_as_tables Callback: displayCexTables(1, 1);
      mask DialogControl Display_counter_example_as_HTML_tables Prompt: Display counter example as HTML tables
      mask DialogControl Display_counter_example_as_HTML_tables Callback: displayCexHtmlTables(1, 1);
      mask DialogControl Generate_an_outer_model_for_the_counter_example Prompt: Generate an outer model for the counter example
      mask DialogControl Generate_an_outer_model_for_the_counter_example Callback: generateModelWithSignalBuilders(1, 1, 2);
      mask DialogControl Generate_an_inner_model_for_the_counter_example Prompt: Generate an inner model for the counter example
      mask DialogControl Generate_an_inner_model_for_the_counter_example Callback: generateModelWithSignalBuilders(1, 1, 1);
  assume : Subsystem  TreatAsAtomicUnit=on  mask(ContractAssumeBlock){ContractBlockType=ContractAssumeBlock}
      mask init:
      | set_param(gcb, 'LinkStatus', 'none');
      mask DialogControl DescTextVar Prompt: Assume block
  lowSpeedWarningTrue_operator : RelationalOperator  Operator===  OutDataTypeStr=boolean  RndMeth=Simplest
  spec122_operator : RelationalOperator  Operator=>  OutDataTypeStr=boolean  RndMeth=Simplest
  spec122_rhs_2 : Constant  Value=0.0  OutDataTypeStr=double
  spec139_operator : Subsystem  TreatAsAtomicUnit=on
  spec156_operator : Subsystem  TreatAsAtomicUnit=on
  spec170_operator : Subsystem  TreatAsAtomicUnit=on
  sqrtOfWeight_sqrt_call : Sqrt  SaturateOnIntegerOverflow=on
  validator : M-S-Function  LoadFcn=saveValidatorParameters(gcb);  InitFcn=contractBeforeSimulation();  StopFcn=contractAfterSimulation();  FunctionName=contract  mask(ContractValidatorBlock){assumePorts=1, guaranteePorts=3, modePorts=0, ContractBlockType=ContractValidatorBlock, createInportsCheckbox=off}
      mask prompts: assumePorts "Assume ports     :"; guaranteePorts "Guarantee ports :"; modePorts "Mode ports        :"; createInportsCheckbox "Create inports and connect them automatically"
      mask init:
      | set_param(gcb,'LinkStatus','none');
      | contract_callback('inputs_callback',gcb);
      mask DialogControl DescTextVar Prompt: The validator block implements the following logic: <br> <br> <b>Sofar</b>(assume<sub>1</sub> <b>&#8743;</b> assume<sub>2</sub> <b>&#8743;</b> ... assume<sub>k</sub>) <b>&rarr;</b> (guarantee<sub>1</sub> <b>&#8743;</b> guarantee<sub>2</sub> <b>&#8743;</b> ... guarantee<sub>m</sub> <b>&#8743;</b>  mode<sub>1</sub> <b>&#8743;</b> mode<sub>2</sub> <b>&#8743;</b> ... <b>&#8743;</b> mode<sub>n</sub> )<br> where mode<sub>i</sub> = require<sub>i</sub> <b>&rarr;</b> ensure<sub>i</sub>
      mask Display:
      | color('black');
      | port_label('input',1,'assume');
      | port_label('input',2,'guarantee');
      | port_label('input',3,'guarantee');
      | port_label('input',4,'guarantee');
      | port_label('output',1,'valid');
  xxSWIMSpec_10_operator : RelationalOperator  Operator===  OutDataTypeStr=boolean  RndMeth=Simplest
  xxSWIMSpec_11_operator : RelationalOperator  Operator===  OutDataTypeStr=boolean  RndMeth=Simplest
  xxSWIMSpec_12_rhs : Constant  Value=1.0  OutDataTypeStr=double
  xxSWIMSpec_13_rhs : Constant  Value=0  OutDataTypeStr=Inherit: Inherit via back propagation
  xxSWIMSpec_14_rhs : Constant  OutDataTypeStr=Inherit: Inherit via back propagation
  xxSWIMSpec_1_operator : RelationalOperator  Operator=<  OutDataTypeStr=boolean  RndMeth=Simplest
  xxSWIMSpec_2_operator : RelationalOperator  Operator===  OutDataTypeStr=boolean  RndMeth=Simplest
  xxSWIMSpec_2_rhs_2 : Constant  Value=1.0  OutDataTypeStr=double
  xxSWIMSpec_3_operator : Logic  AllPortsSameDT=off  OutDataTypeStr=boolean
  xxSWIMSpec_4_operator : Product  OutDataTypeStr=double
  xxSWIMSpec_4_rhs_1 : Constant  Value=1.33694  OutDataTypeStr=double
  xxSWIMSpec_5_operator : Sum  OutDataTypeStr=double
  xxSWIMSpec_5_rhs_2 : Constant  Value=10.0  OutDataTypeStr=double
  xxSWIMSpec_6_operator : RelationalOperator  Operator===  OutDataTypeStr=boolean  RndMeth=Simplest
  xxSWIMSpec_7_operator : RelationalOperator  Operator===  OutDataTypeStr=boolean  RndMeth=Simplest
  xxSWIMSpec_8_operator : Product  OutDataTypeStr=double
  xxSWIMSpec_8_rhs_1 : Constant  Value=1.25921  OutDataTypeStr=double
  xxSWIMSpec_9_operator : Sum  OutDataTypeStr=double
  xxSWIMSpec_9_rhs_2 : Constant  Value=10.0  OutDataTypeStr=double
  valid : Outport
  wires:
  validator/1 -> valid/1
  xxSWIMSpec_9_rhs_2/1 -> xxSWIMSpec_9_operator/2
  xxSWIMSpec_8_operator/1 -> xxSWIMSpec_9_operator/1
  xxSWIMSpec_8_rhs_1/1 -> xxSWIMSpec_8_operator/1
  xxSWIMSpec_14_rhs/1 -> xxSWIMSpec_7_operator/2
  xxSWIMSpec_5_operator/1 -> xxSWIMSpec_6_operator/2
  xxSWIMSpec_5_rhs_2/1 -> xxSWIMSpec_5_operator/2
  xxSWIMSpec_4_operator/1 -> xxSWIMSpec_5_operator/1
  xxSWIMSpec_4_rhs_1/1 -> xxSWIMSpec_4_operator/1
  xxSWIMSpec_1_operator/1 -> xxSWIMSpec_3_operator/2
  xxSWIMSpec_2_operator/1 -> xxSWIMSpec_3_operator/1
  xxSWIMSpec_2_rhs_2/1 -> xxSWIMSpec_2_operator/2
  SWIMSpec_lowSpeedWarningAllowed/1 -> xxSWIMSpec_2_operator/1
  SWIMSpec_warningTrigForMinPress/1 -> xxSWIMSpec_1_operator/2
  SWIMSpec_vehAirPress/1 -> xxSWIMSpec_1_operator/1
  xxSWIMSpec_13_rhs/1 -> xxSWIMSpec_11_operator/2
  xxSWIMSpec_9_operator/1 -> xxSWIMSpec_10_operator/2
  SWIM_minus_002/1(guarantee) -> validator/4
  SWIM_minus_001B/1(guarantee) -> validator/3
  SWIM_minus_001A/1(guarantee) -> validator/2
  assume/1(assume) -> validator/1
  lowSpeedWarningTrue_operator/1 -> spec170_operator/2(B)
  xxSWIMSpec_3_operator/1 -> spec170_operator/1(A)
  xxSWIMSpec_6_operator/1 -> spec156_operator/2(B)
  xxSWIMSpec_7_operator/1 -> spec156_operator/1(A)
  xxSWIMSpec_10_operator/1 -> spec139_operator/2(B)
  xxSWIMSpec_11_operator/1 -> spec139_operator/1(A)
  spec122_rhs_2/1 -> spec122_operator/2
  xxSWIMSpec_12_rhs/1 -> lowSpeedWarningTrue_operator/2
  SWIMSpec_swimGet_agcasLowSpeedWarn/1 -> lowSpeedWarningTrue_operator/1
  spec170_operator/1(A_equal__equal__gt_B) -> SWIM_minus_002/1(In1)
  spec156_operator/1(A_equal__equal__gt_B) -> SWIM_minus_001B/1(In1)
  spec139_operator/1(A_equal__equal__gt_B) -> SWIM_minus_001A/1(In1)
  spec122_operator/1 -> assume/1(In1)
  SWIMSpec_weight/1 -> sqrtOfWeight_sqrt_call/1, spec122_operator/1
  SWIMSpec_CalAirspeedMin/1 -> xxSWIMSpec_6_operator/1, xxSWIMSpec_10_operator/1
  SWIMSpec_storeCat/1 -> xxSWIMSpec_7_operator/1, xxSWIMSpec_11_operator/1
  sqrtOfWeight_sqrt_call/1 -> xxSWIMSpec_8_operator/2, xxSWIMSpec_4_operator/2

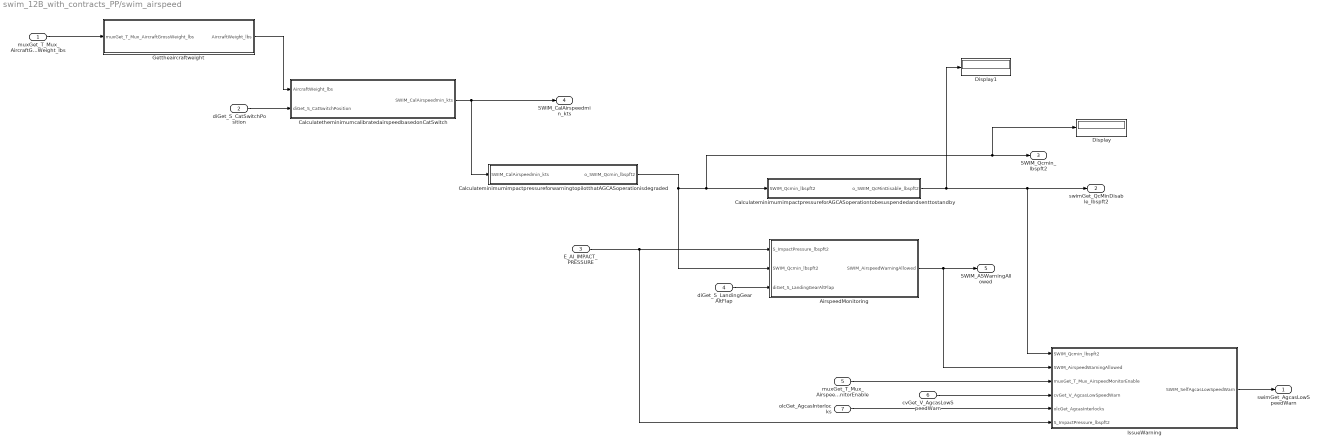
== system swim_12B_with_contracts_PP/swim_airspeed ==
  muxGet_T_Mux_AircraftGrossWeight_lbs : Inport
  diGet_S_CatSwitchPosition : Inport  Port=2
  E_AI_IMPACT_PRESSURE : Inport  Port=3
  diGet_S_LandingGearAltFlap : Inport  Port=4
  muxGet_T_Mux_AirspeedMonitorEnable : Inport  Port=5
  cvGet_V_AgcasLowSpeedWarn : Inport  Port=6
  olcGet_AgcasInterlocks : Inport  Port=7
  AirspeedMonitoring : Subsystem  TreatAsAtomicUnit=on
  CalculateminimumimpactpressureforAGCASoperationtobesuspendedandsenttostandby : Subsystem  TreatAsAtomicUnit=on
  CalculateminimumimpactpressureforwarningtopilotthatAGCASoperationisdegraded : Subsystem  TreatAsAtomicUnit=on
  CalculatetheminimumcalibratedairspeedbasedonCatSwitch : Subsystem  TreatAsAtomicUnit=on
  Display : Display
  Display1 : Display
  Gettheaircraftweight : Subsystem  TreatAsAtomicUnit=on
  IssueWarning : Subsystem  TreatAsAtomicUnit=on
  swimGet_AgcasLowSpeedWarn : Outport  VectorParamsAs1DForOutWhenUnconnected=off
  swimGet_QcMinDisable_lbspft2 : Outport  Port=2  VectorParamsAs1DForOutWhenUnconnected=off
  SWIM_Qcmin_lbspft2 : Outport  Port=3  VectorParamsAs1DForOutWhenUnconnected=off
  SWIM_CalAirspeedmin_kts : Outport  Port=4  VectorParamsAs1DForOutWhenUnconnected=off
  SWIM_ASWarningAllowed : Outport  Port=5  VectorParamsAs1DForOutWhenUnconnected=off
  wires:
  muxGet_T_Mux_AircraftGrossWeight_lbs/1 -> Gettheaircraftweight/1(muxGet_T_Mux_AircraftGrossWeight_lbs)
  diGet_S_CatSwitchPosition/1 -> CalculatetheminimumcalibratedairspeedbasedonCatSwitch/2(diGet_S_CatSwitchPosition)
  Gettheaircraftweight/1(AircraftWeight_lbs) -> CalculatetheminimumcalibratedairspeedbasedonCatSwitch/1(AircraftWeight_lbs)
  CalculatetheminimumcalibratedairspeedbasedonCatSwitch/1(SWIM_CalAirspeedmin_kts) -> CalculateminimumimpactpressureforwarningtopilotthatAGCASoperationisdegraded/1(SWIM_CalAirspeedmin_kts), SWIM_CalAirspeedmin_kts/1
  E_AI_IMPACT_PRESSURE/1 -> IssueWarning/6(S_ImpactPressure_lbspft2), AirspeedMonitoring/1(S_ImpactPressure_lbspft2)
  diGet_S_LandingGearAltFlap/1 -> AirspeedMonitoring/3(diGet_S_LandingGearAltFlap)
  IssueWarning/1(SWIM_SelfAgcasLowSpeedWarn) -> swimGet_AgcasLowSpeedWarn/1
  muxGet_T_Mux_AirspeedMonitorEnable/1 -> IssueWarning/3(muxGet_T_Mux_AirspeedMonitorEnable)
  cvGet_V_AgcasLowSpeedWarn/1 -> IssueWarning/4(cvGet_V_AgcasLowSpeedWarn)
  olcGet_AgcasInterlocks/1 -> IssueWarning/5(olcGet_AgcasInterlocks)
  CalculateminimumimpactpressureforAGCASoperationtobesuspendedandsenttostandby/1(o_SWIM_QcMinDisable_lbspft2) -> Display1/1, IssueWarning/1(SWIM_Qcmin_lbspft2), swimGet_QcMinDisable_lbspft2/1
  AirspeedMonitoring/1(SWIM_AirspeedWarningAllowed) -> IssueWarning/2(SWIM_AirspeedWarningAllowed), SWIM_ASWarningAllowed/1
  CalculateminimumimpactpressureforwarningtopilotthatAGCASoperationisdegraded/1(o_SWIM_Qcmin_lbspft2) -> AirspeedMonitoring/2(SWIM_Qcmin_lbspft2), Display/1, SWIM_Qcmin_lbspft2/1, CalculateminimumimpactpressureforAGCASoperationtobesuspendedandsenttostandby/1(SWIM_Qcmin_lbspft2)

== system swim_12B_with_contracts_PP/swim_12B_SWIMSpec/SWIM_minus_001A ==
  In1 : Inport
  guarantee : Outport  OutDataTypeStr=boolean
  wires:
  In1/1 -> guarantee/1

== system swim_12B_with_contracts_PP/swim_12B_SWIMSpec/SWIM_minus_001B ==
  In1 : Inport
  guarantee : Outport  OutDataTypeStr=boolean
  wires:
  In1/1 -> guarantee/1

== system swim_12B_with_contracts_PP/swim_12B_SWIMSpec/SWIM_minus_002 ==
  In1 : Inport
  guarantee : Outport  OutDataTypeStr=boolean
  wires:
  In1/1 -> guarantee/1

== system swim_12B_with_contracts_PP/swim_12B_SWIMSpec/assume ==
  In1 : Inport
  assume : Outport  OutDataTypeStr=boolean
  wires:
  In1/1 -> assume/1

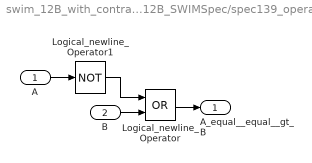
== system swim_12B_with_contracts_PP/swim_12B_SWIMSpec/spec139_operator ==
  A : Inport
  B : Inport  Port=2
  Logical_newline_Operator : Logic  Operator=OR  AllPortsSameDT=off  OutDataTypeStr=boolean
  Logical_newline_Operator1 : Logic  Operator=NOT  AllPortsSameDT=off  OutDataTypeStr=boolean
  A_equal__equal__gt_B : Outport  VectorParamsAs1DForOutWhenUnconnected=off
  wires:
  B/1 -> Logical_newline_Operator/2
  A/1 -> Logical_newline_Operator1/1
  Logical_newline_Operator/1 -> A_equal__equal__gt_B/1
  Logical_newline_Operator1/1 -> Logical_newline_Operator/1

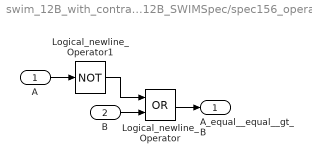
== system swim_12B_with_contracts_PP/swim_12B_SWIMSpec/spec156_operator ==
  A : Inport
  B : Inport  Port=2
  Logical_newline_Operator : Logic  Operator=OR  AllPortsSameDT=off  OutDataTypeStr=boolean
  Logical_newline_Operator1 : Logic  Operator=NOT  AllPortsSameDT=off  OutDataTypeStr=boolean
  A_equal__equal__gt_B : Outport  VectorParamsAs1DForOutWhenUnconnected=off
  wires:
  B/1 -> Logical_newline_Operator/2
  A/1 -> Logical_newline_Operator1/1
  Logical_newline_Operator/1 -> A_equal__equal__gt_B/1
  Logical_newline_Operator1/1 -> Logical_newline_Operator/1

== system swim_12B_with_contracts_PP/swim_12B_SWIMSpec/spec170_operator ==
  A : Inport
  B : Inport  Port=2
  Logical_newline_Operator : Logic  Operator=OR  AllPortsSameDT=off  OutDataTypeStr=boolean
  Logical_newline_Operator1 : Logic  Operator=NOT  AllPortsSameDT=off  OutDataTypeStr=boolean
  A_equal__equal__gt_B : Outport  VectorParamsAs1DForOutWhenUnconnected=off
  wires:
  B/1 -> Logical_newline_Operator/2
  A/1 -> Logical_newline_Operator1/1
  Logical_newline_Operator/1 -> A_equal__equal__gt_B/1
  Logical_newline_Operator1/1 -> Logical_newline_Operator/1

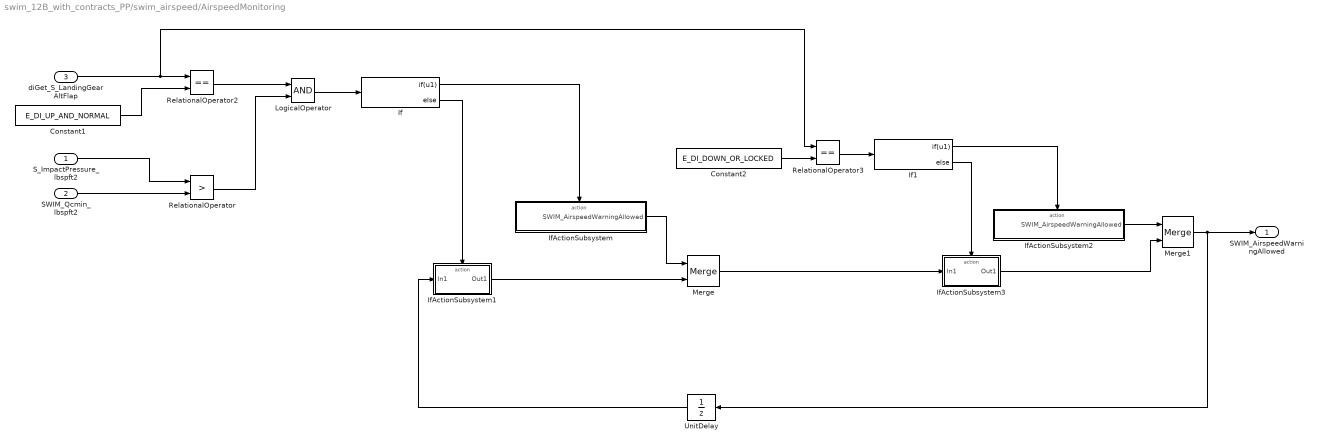
== system swim_12B_with_contracts_PP/swim_airspeed/AirspeedMonitoring ==
  S_ImpactPressure_lbspft2 : Inport
  SWIM_Qcmin_lbspft2 : Inport  Port=2
  diGet_S_LandingGearAltFlap : Inport  Port=3
  Constant1 : Constant  Value=E_DI_UP_AND_NORMAL
  Constant2 : Constant  Value=E_DI_DOWN_OR_LOCKED
  If : If  IfExpression=u1
  If1 : If  IfExpression=u1
  IfActionSubsystem : Subsystem  TreatAsAtomicUnit=on
  IfActionSubsystem1 : Subsystem  TreatAsAtomicUnit=on
  IfActionSubsystem2 : Subsystem  TreatAsAtomicUnit=on
  IfActionSubsystem3 : Subsystem  TreatAsAtomicUnit=on
  LogicalOperator : Logic  AllPortsSameDT=off  OutDataTypeStr=boolean
  Merge : Merge
  Merge1 : Merge
  RelationalOperator : RelationalOperator  Operator=>  OutDataTypeStr=boolean  RndMeth=Nearest
  RelationalOperator2 : RelationalOperator  Operator===  OutDataTypeStr=boolean  RndMeth=Nearest
  RelationalOperator3 : RelationalOperator  Operator===  OutDataTypeStr=boolean  RndMeth=Nearest
  UnitDelay : UnitDelay  InitialCondition=E_SWIM_NOT_ALLOWED  SampleTime=-1  HasFrameUpgradeWarning=on
  SWIM_AirspeedWarningAllowed : Outport  VectorParamsAs1DForOutWhenUnconnected=off
  wires:
  S_ImpactPressure_lbspft2/1 -> RelationalOperator/1
  SWIM_Qcmin_lbspft2/1 -> RelationalOperator/2
  diGet_S_LandingGearAltFlap/1 -> RelationalOperator3/1, RelationalOperator2/1
  Constant1/1 -> RelationalOperator2/2
  If/1 -> IfActionSubsystem/Action
  If/2 -> IfActionSubsystem1/Action
  IfActionSubsystem/1(SWIM_AirspeedWarningAllowed) -> Merge/1
  IfActionSubsystem1/1(Out1) -> Merge/2
  Constant2/1 -> RelationalOperator3/2
  RelationalOperator3/1 -> If1/1
  RelationalOperator/1 -> LogicalOperator/2
  RelationalOperator2/1 -> LogicalOperator/1
  LogicalOperator/1 -> If/1
  If1/1 -> IfActionSubsystem2/Action
  If1/2 -> IfActionSubsystem3/Action
  IfActionSubsystem2/1(SWIM_AirspeedWarningAllowed) -> Merge1/1
  IfActionSubsystem3/1(Out1) -> Merge1/2
  Merge/1 -> IfActionSubsystem3/1(In1)
  Merge1/1 -> UnitDelay/1, SWIM_AirspeedWarningAllowed/1
  UnitDelay/1 -> IfActionSubsystem1/1(In1)

== system swim_12B_with_contracts_PP/swim_airspeed/CalculateminimumimpactpressureforAGCASoperationtobesuspendedandsenttostandby ==
  SWIM_Qcmin_lbspft2 : Inport
  Constant : Constant  Value=-28.72
  Sum : Sum  Inputs=|++
  o_SWIM_QcMinDisable_lbspft2 : Outport  VectorParamsAs1DForOutWhenUnconnected=off
  wires:
  SWIM_Qcmin_lbspft2/1 -> Sum/1
  Constant/1 -> Sum/2
  Sum/1 -> o_SWIM_QcMinDisable_lbspft2/1

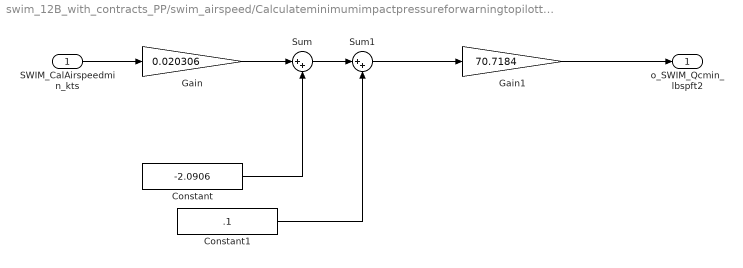
== system swim_12B_with_contracts_PP/swim_airspeed/CalculateminimumimpactpressureforwarningtopilotthatAGCASoperationisdegraded ==
  SWIM_CalAirspeedmin_kts : Inport
  Constant : Constant  Value=-2.0906
  Constant1 : Constant  Value=.1
  Gain : Gain  Gain=0.020306
  Gain1 : Gain  Gain=70.7184
  Sum : Sum  Inputs=|++
  Sum1 : Sum  Inputs=|++
  o_SWIM_Qcmin_lbspft2 : Outport  VectorParamsAs1DForOutWhenUnconnected=off
  wires:
  SWIM_CalAirspeedmin_kts/1 -> Gain/1
  Gain/1 -> Sum/1
  Constant/1 -> Sum/2
  Sum/1 -> Sum1/1
  Constant1/1 -> Sum1/2
  Sum1/1 -> Gain1/1
  Gain1/1 -> o_SWIM_Qcmin_lbspft2/1

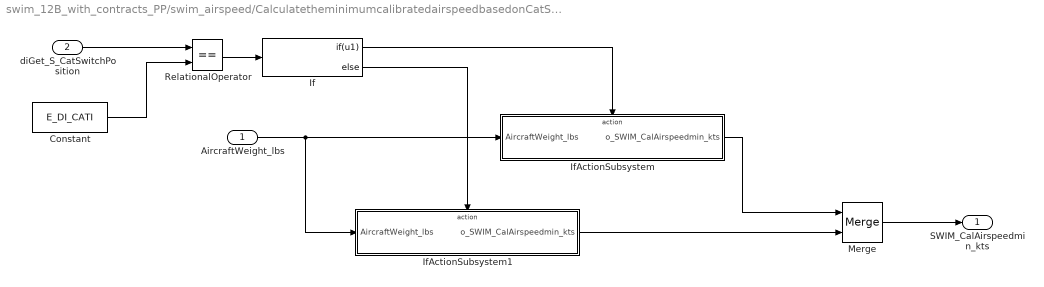
== system swim_12B_with_contracts_PP/swim_airspeed/CalculatetheminimumcalibratedairspeedbasedonCatSwitch ==
  AircraftWeight_lbs : Inport
  diGet_S_CatSwitchPosition : Inport  Port=2
  Constant : Constant  Value=E_DI_CATI
  If : If  IfExpression=u1
  IfActionSubsystem : Subsystem  TreatAsAtomicUnit=on
  IfActionSubsystem1 : Subsystem  TreatAsAtomicUnit=on
  Merge : Merge
  RelationalOperator : RelationalOperator  Operator===  OutDataTypeStr=boolean  RndMeth=Nearest
  SWIM_CalAirspeedmin_kts : Outport  VectorParamsAs1DForOutWhenUnconnected=off
  wires:
  If/1 -> IfActionSubsystem/Action
  If/2 -> IfActionSubsystem1/Action
  IfActionSubsystem/1(o_SWIM_CalAirspeedmin_kts) -> Merge/1
  IfActionSubsystem1/1(o_SWIM_CalAirspeedmin_kts) -> Merge/2
  Merge/1 -> SWIM_CalAirspeedmin_kts/1
  AircraftWeight_lbs/1 -> IfActionSubsystem/1(AircraftWeight_lbs), IfActionSubsystem1/1(AircraftWeight_lbs)
  Constant/1 -> RelationalOperator/2
  diGet_S_CatSwitchPosition/1 -> RelationalOperator/1
  RelationalOperator/1 -> If/1

== system swim_12B_with_contracts_PP/swim_airspeed/Gettheaircraftweight ==
  muxGet_T_Mux_AircraftGrossWeight_lbs : Inport
  AircraftWeight_lbs : Outport  VectorParamsAs1DForOutWhenUnconnected=off
  wires:
  muxGet_T_Mux_AircraftGrossWeight_lbs/1 -> AircraftWeight_lbs/1

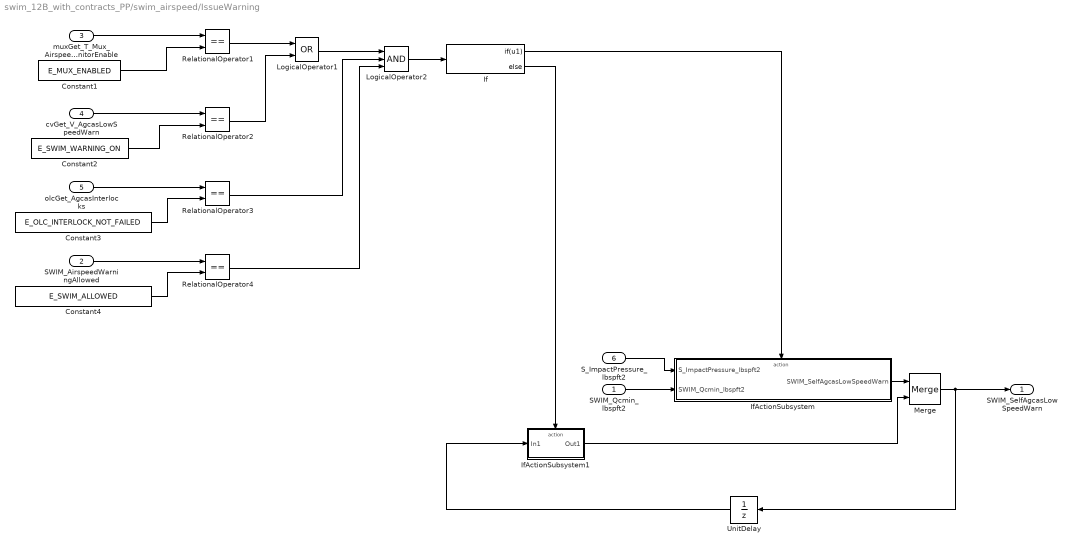
== system swim_12B_with_contracts_PP/swim_airspeed/IssueWarning ==
  SWIM_Qcmin_lbspft2 : Inport
  SWIM_AirspeedWarningAllowed : Inport  Port=2
  muxGet_T_Mux_AirspeedMonitorEnable : Inport  Port=3
  cvGet_V_AgcasLowSpeedWarn : Inport  Port=4
  olcGet_AgcasInterlocks : Inport  Port=5
  S_ImpactPressure_lbspft2 : Inport  Port=6
  Constant1 : Constant  Value=E_MUX_ENABLED
  Constant2 : Constant  Value=E_SWIM_WARNING_ON
  Constant3 : Constant  Value=E_OLC_INTERLOCK_NOT_FAILED
  Constant4 : Constant  Value=E_SWIM_ALLOWED
  If : If  IfExpression=u1
  IfActionSubsystem : Subsystem  TreatAsAtomicUnit=on
  IfActionSubsystem1 : Subsystem  TreatAsAtomicUnit=on
  LogicalOperator1 : Logic  Operator=OR  AllPortsSameDT=off  OutDataTypeStr=boolean
  LogicalOperator2 : Logic  Inputs=3  AllPortsSameDT=off  OutDataTypeStr=boolean
  Merge : Merge
  RelationalOperator{1..4} (4 alike) : RelationalOperator  Operator===  OutDataTypeStr=boolean  RndMeth=Nearest
  UnitDelay : UnitDelay  InitialCondition=E_SWIM_WARNING_OFF  SampleTime=-1  HasFrameUpgradeWarning=on
  SWIM_SelfAgcasLowSpeedWarn : Outport  VectorParamsAs1DForOutWhenUnconnected=off
  wires:
  muxGet_T_Mux_AirspeedMonitorEnable/1 -> RelationalOperator1/1
  cvGet_V_AgcasLowSpeedWarn/1 -> RelationalOperator2/1
  Constant2/1 -> RelationalOperator2/2
  Constant1/1 -> RelationalOperator1/2
  olcGet_AgcasInterlocks/1 -> RelationalOperator3/1
  Constant3/1 -> RelationalOperator3/2
  SWIM_AirspeedWarningAllowed/1 -> RelationalOperator4/1
  Constant4/1 -> RelationalOperator4/2
  RelationalOperator1/1 -> LogicalOperator1/1
  RelationalOperator2/1 -> LogicalOperator1/2
  LogicalOperator1/1 -> LogicalOperator2/1
  RelationalOperator3/1 -> LogicalOperator2/2
  RelationalOperator4/1 -> LogicalOperator2/3
  LogicalOperator2/1 -> If/1
  If/1 -> IfActionSubsystem/Action
  If/2 -> IfActionSubsystem1/Action
  SWIM_Qcmin_lbspft2/1 -> IfActionSubsystem/2(SWIM_Qcmin_lbspft2)
  IfActionSubsystem/1(SWIM_SelfAgcasLowSpeedWarn) -> Merge/1
  Merge/1 -> UnitDelay/1, SWIM_SelfAgcasLowSpeedWarn/1
  IfActionSubsystem1/1(Out1) -> Merge/2
  UnitDelay/1 -> IfActionSubsystem1/1(In1)
  S_ImpactPressure_lbspft2/1 -> IfActionSubsystem/1(S_ImpactPressure_lbspft2)

== system swim_12B_with_contracts_PP/swim_airspeed/AirspeedMonitoring/IfActionSubsystem ==
  ActionPort : ActionPort  ActionPortLabel=if(u1)
  Constant : Constant  Value=E_SWIM_ALLOWED
  SWIM_AirspeedWarningAllowed : Outport  VectorParamsAs1DForOutWhenUnconnected=off
  wires:
  Constant/1 -> SWIM_AirspeedWarningAllowed/1

== system swim_12B_with_contracts_PP/swim_airspeed/AirspeedMonitoring/IfActionSubsystem1 ==
  In1 : Inport
  ActionPort : ActionPort  ActionPortLabel=else
  Out1 : Outport  VectorParamsAs1DForOutWhenUnconnected=off
  wires:
  In1/1 -> Out1/1

== system swim_12B_with_contracts_PP/swim_airspeed/AirspeedMonitoring/IfActionSubsystem2 ==
  ActionPort : ActionPort  ActionPortLabel=if(u1)
  Constant : Constant  Value=E_SWIM_NOT_ALLOWED
  SWIM_AirspeedWarningAllowed : Outport  VectorParamsAs1DForOutWhenUnconnected=off
  wires:
  Constant/1 -> SWIM_AirspeedWarningAllowed/1

== system swim_12B_with_contracts_PP/swim_airspeed/AirspeedMonitoring/IfActionSubsystem3 ==
  In1 : Inport
  ActionPort : ActionPort  ActionPortLabel=else
  Out1 : Outport  VectorParamsAs1DForOutWhenUnconnected=off
  wires:
  In1/1 -> Out1/1

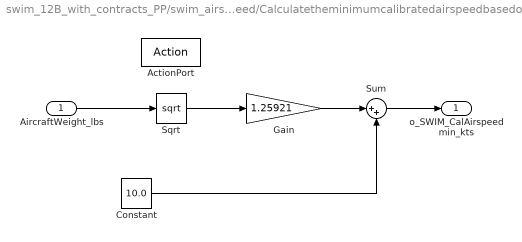
== system swim_12B_with_contracts_PP/swim_airspeed/CalculatetheminimumcalibratedairspeedbasedonCatSwitch/IfActionSubsystem ==
  AircraftWeight_lbs : Inport
  ActionPort : ActionPort  ActionPortLabel=if(u1)
  Constant : Constant  Value=10.0
  Gain : Gain  Gain=1.25921
  Sqrt : Sqrt  SaturateOnIntegerOverflow=on
  Sum : Sum  Inputs=|++
  o_SWIM_CalAirspeedmin_kts : Outport  VectorParamsAs1DForOutWhenUnconnected=off
  wires:
  AircraftWeight_lbs/1 -> Sqrt/1
  Gain/1 -> Sum/1
  Constant/1 -> Sum/2
  Sum/1 -> o_SWIM_CalAirspeedmin_kts/1
  Sqrt/1 -> Gain/1

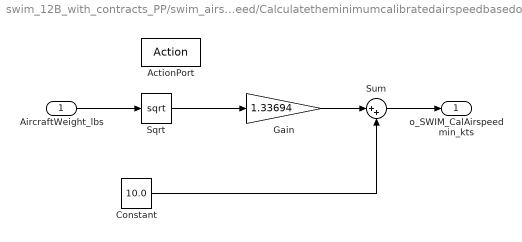
== system swim_12B_with_contracts_PP/swim_airspeed/CalculatetheminimumcalibratedairspeedbasedonCatSwitch/IfActionSubsystem1 ==
  AircraftWeight_lbs : Inport
  ActionPort : ActionPort  ActionPortLabel=else
  Constant : Constant  Value=10.0
  Gain : Gain  Gain=1.33694
  Sqrt : Sqrt  SaturateOnIntegerOverflow=on
  Sum : Sum  Inputs=|++
  o_SWIM_CalAirspeedmin_kts : Outport  VectorParamsAs1DForOutWhenUnconnected=off
  wires:
  Sum/1 -> o_SWIM_CalAirspeedmin_kts/1
  Constant/1 -> Sum/2
  Gain/1 -> Sum/1
  AircraftWeight_lbs/1 -> Sqrt/1
  Sqrt/1 -> Gain/1

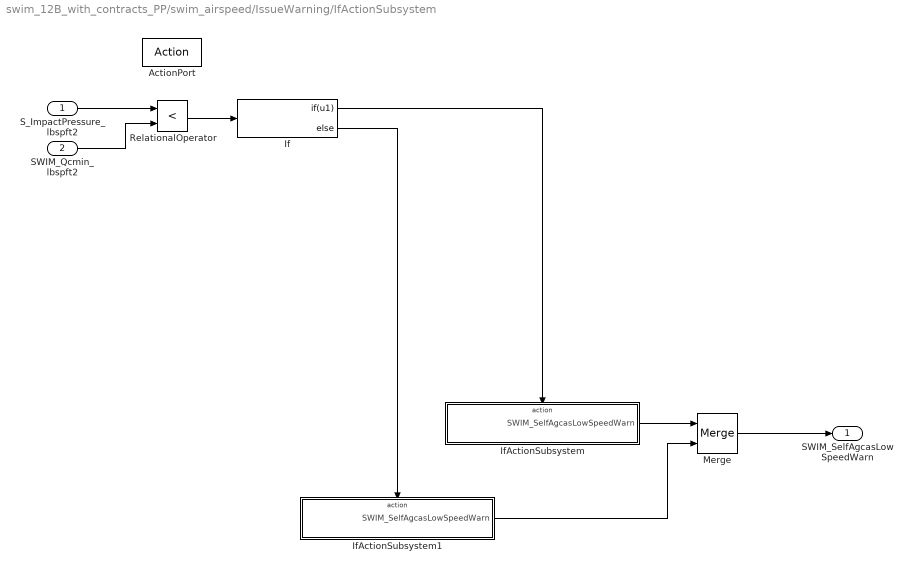
== system swim_12B_with_contracts_PP/swim_airspeed/IssueWarning/IfActionSubsystem ==
  S_ImpactPressure_lbspft2 : Inport
  SWIM_Qcmin_lbspft2 : Inport  Port=2
  ActionPort : ActionPort  ActionPortLabel=if(u1)
  If : If  IfExpression=u1
  IfActionSubsystem : Subsystem  TreatAsAtomicUnit=on
  IfActionSubsystem1 : Subsystem  TreatAsAtomicUnit=on
  Merge : Merge
  RelationalOperator : RelationalOperator  Operator=<  OutDataTypeStr=boolean  RndMeth=Nearest
  SWIM_SelfAgcasLowSpeedWarn : Outport  VectorParamsAs1DForOutWhenUnconnected=off
  wires:
  S_ImpactPressure_lbspft2/1 -> RelationalOperator/1
  SWIM_Qcmin_lbspft2/1 -> RelationalOperator/2
  If/1 -> IfActionSubsystem/Action
  RelationalOperator/1 -> If/1
  Merge/1 -> SWIM_SelfAgcasLowSpeedWarn/1
  IfActionSubsystem/1(SWIM_SelfAgcasLowSpeedWarn) -> Merge/1
  IfActionSubsystem1/1(SWIM_SelfAgcasLowSpeedWarn) -> Merge/2
  If/2 -> IfActionSubsystem1/Action

== system swim_12B_with_contracts_PP/swim_airspeed/IssueWarning/IfActionSubsystem1 ==
  In1 : Inport
  ActionPort : ActionPort  ActionPortLabel=else
  Out1 : Outport  VectorParamsAs1DForOutWhenUnconnected=off
  wires:
  In1/1 -> Out1/1

== system swim_12B_with_contracts_PP/swim_airspeed/IssueWarning/IfActionSubsystem/IfActionSubsystem ==
  ActionPort : ActionPort  ActionPortLabel=if(u1)
  Constant : Constant  Value=E_SWIM_WARNING_ON
  SWIM_SelfAgcasLowSpeedWarn : Outport  VectorParamsAs1DForOutWhenUnconnected=off
  wires:
  Constant/1 -> SWIM_SelfAgcasLowSpeedWarn/1

== system swim_12B_with_contracts_PP/swim_airspeed/IssueWarning/IfActionSubsystem/IfActionSubsystem1 ==
  ActionPort : ActionPort  ActionPortLabel=else
  Constant : Constant  Value=E_SWIM_WARNING_OFF
  SWIM_SelfAgcasLowSpeedWarn : Outport  VectorParamsAs1DForOutWhenUnconnected=off
  wires:
  Constant/1 -> SWIM_SelfAgcasLowSpeedWarn/1
